simulink model "borrador_modelo_completo"  (R2016b)
settings: Solver=VariableStepAuto  StartTime=0.0  StopTime=10.0  RelTol=1e-3
values from neighbouring files (symbols this model uses):
  Rs = 1.02    [c4ModeloCompleto_var.m]
settings Model: Creator=agustin  LastModifiedBy=agustin

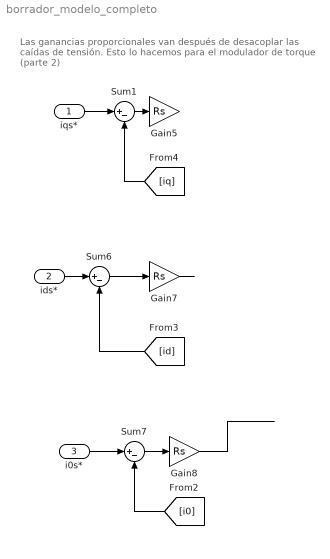
== system borrador_modelo_completo ==
  note: Las ganancias proporcionales van después de desacoplar las caídas de tensión.
      | Esto lo hacemos para el modulador de torque (parte 2)
  iqs* : Inport
  ids* : Inport  Port=2
  i0s* : Inport  Port=3
  Gain5 : Gain  Gain=Rs
  Gain7 : Gain  Gain=Rs
  Gain8 : Gain  Gain=Rs
  Sum1 : Sum  Inputs=|+-
  Sum6 : Sum  Inputs=|+-
  Sum7 : Sum  Inputs=|+-
  wires:
  iqs*/1 -> Sum1/1
  Sum1/1 -> Gain5/1
  [iq] -> Sum1/2
  Gain7/1 -> ?
  ids*/1 -> Sum6/1
  Sum6/1 -> Gain7/1
  [id] -> Sum6/2
  Gain8/1 -> ?
  i0s*/1 -> Sum7/1
  Sum7/1 -> Gain8/1
  [i0] -> Sum7/2
